simulink model "Figure_2_4_TP_Modulation_phase_quadrature"  (R2020a)
settings: Solver=FixedStepDiscrete  StartTime=0.0  StopTime=inf  RelTol=1e-3
libraries: dspsrcs4 x5, commutil2 x4, simulink x3, commrandsrc3 x2, commfilt2 x2, commsink2 x1
settings Model: Creator=iba  LastModifiedBy=iba

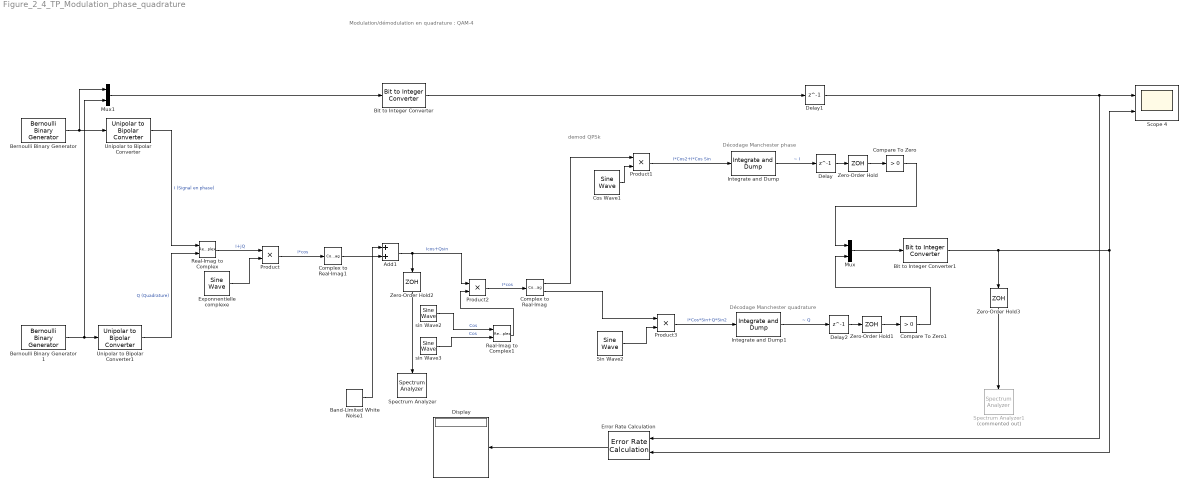
== system Figure_2_4_TP_Modulation_phase_quadrature ==
  note: Décodage Manchester phase
  note: Décodage Manchester quadrature
  note: demod QPSk
  note: Modulation/démodulation en quadrature : QAM-4
  Add1 : Sum
  Band-Limited White Noise1 : simulink/Sources/Band-Limited White Noise  Cov=1e-3  Ts=0.1  seed=1
  "Bernoulli Binary Generator " : commrandsrc3/Bernoulli Binary Generator  ProbabilityOfZero=0.5  SeedSource=Parameter  Seed=61  SampleTime=1  SamplesPerFrame=1  OutputDataType=double  SimulateUsing=Interpreted execution
  Bernoulli Binary Generator 1 : commrandsrc3/Bernoulli Binary Generator  ProbabilityOfZero=0.5  SeedSource=Parameter  Seed=23  SampleTime=1  SamplesPerFrame=1  OutputDataType=double  SimulateUsing=Interpreted execution
  Bit to Integer Converter : commutil2/Bit to Integer Converter  nbits=2  bitOrder=MSB first  signedOutputValues=Unsigned  outDtype=double  outDtypeSigned=Inherit via internal rule
  Bit to Integer Converter1 : commutil2/Bit to Integer Converter  nbits=2  bitOrder=MSB first  signedOutputValues=Unsigned  outDtype=double  outDtypeSigned=Inherit via internal rule
  Compare To Zero : simulink/Logic and Bit Operations/Compare To Zero  relop=>  OutDataTypeStr=boolean
  Compare To Zero1 : simulink/Logic and Bit Operations/Compare To Zero  relop=>  OutDataTypeStr=boolean
  Complex to Real-Imag : ComplexToRealImag
  Complex to Real-Imag1 : ComplexToRealImag  Output=Real
  Cos Wave1 : dspsrcs4/Sine Wave  Amplitude=1  Frequency=5  Phase=pi/2  SampleMode=Discrete  OutComplex=Real  CompMethod=Trigonometric fcn  TableSize=Speed  SampleTime=1/100  SamplesPerFrame=1  ResetState=Restart at time zero  OutputFrames=off  dataType=double  wordLen=16  udDataType=sfix(16)  fracBitsMode=Best precision  numFracBits=15  OutDataTypeStr=double  LastOutDataTypeStr=double
  Delay : Delay  DelayLength=1  InitialCondition=0
  Delay1 : Delay  DelayLength=1  InitialCondition=0
  Delay2 : Delay  DelayLength=1  InitialCondition=0
  Display : Display
  Error Rate Calculation : commsink2/Error Rate Calculation  N=0  st_delay=0  cp_mode=Entire frame  subframe=[]  PMode=Port  WsName=ErrorVec  RsMode2=off  stop=on  numErr=1000  maxBits=1000
  Exponnentielle complexe : dspsrcs4/Sine Wave  Amplitude=exp(1)  Frequency=5  Phase=0  SampleMode=Discrete  OutComplex=Real  CompMethod=Trigonometric fcn  TableSize=Speed  SampleTime=1/100  SamplesPerFrame=1  ResetState=Restart at time zero  OutputFrames=off  dataType=double  wordLen=16  udDataType=sfix(16)  fracBitsMode=Best precision  numFracBits=15  OutDataTypeStr=double  LastOutDataTypeStr=double
  Integrate and Dump : commfilt2/Integrate and Dump  obssamples=100  offsetsamples=0  nodump=on  roundingMode=Floor  overflowMode=off  outputDataTypeStr=Inherit: Same as accumulator  outputLastDataTypeStr=Inherit: Same as accumulator
  Integrate and Dump1 : commfilt2/Integrate and Dump  obssamples=100  offsetsamples=0  nodump=on  roundingMode=Floor  overflowMode=off  outputDataTypeStr=Inherit: Same as accumulator  outputLastDataTypeStr=Inherit: Same as accumulator
  Mux : Mux  Inputs=2
  Mux1 : Mux  Inputs=2
  Product{,1..3} (4 alike) : Product
  Real-Imag to Complex : RealImagToComplex
  Real-Imag to Complex1 : RealImagToComplex
  Scope 4 : Scope  NumInputPorts=2
  Sin Wave2 : dspsrcs4/Sine Wave  Amplitude=1  Frequency=5  Phase=0  SampleMode=Discrete  OutComplex=Real  CompMethod=Trigonometric fcn  TableSize=Speed  SampleTime=1/100  SamplesPerFrame=1  ResetState=Restart at time zero  OutputFrames=off  dataType=double  wordLen=16  udDataType=sfix(16)  fracBitsMode=Best precision  numFracBits=15  OutDataTypeStr=double  LastOutDataTypeStr=double
  Spectrum Analyzer : SpectrumAnalyzer
  Spectrum Analyzer1 : SpectrumAnalyzer  Commented=on
  Unipolar to Bipolar Converter : commutil2/Unipolar to Bipolar Converter  M=2  polarity=Positive  dataType=Inherit via internal rule
  Unipolar to Bipolar Converter1 : commutil2/Unipolar to Bipolar Converter  M=2  polarity=Positive  dataType=Inherit via internal rule
  Zero-Order Hold : ZeroOrderHold
  Zero-Order Hold1 : ZeroOrderHold
  Zero-Order Hold2 : ZeroOrderHold  SampleTime=1/20
  Zero-Order Hold3 : ZeroOrderHold  SampleTime=1/20
  sin Wave2 : dspsrcs4/Sine Wave  Amplitude=1  Frequency=5  Phase=0  SampleMode=Discrete  OutComplex=Real  CompMethod=Trigonometric fcn  TableSize=Speed  SampleTime=1/100  SamplesPerFrame=1  ResetState=Restart at time zero  OutputFrames=off  dataType=double  wordLen=16  udDataType=sfix(16)  fracBitsMode=Best precision  numFracBits=15  OutDataTypeStr=double  LastOutDataTypeStr=double
  sin Wave3 : dspsrcs4/Sine Wave  Amplitude=1  Frequency=5  Phase=0  SampleMode=Discrete  OutComplex=Real  CompMethod=Trigonometric fcn  TableSize=Speed  SampleTime=1/100  SamplesPerFrame=1  ResetState=Restart at time zero  OutputFrames=off  dataType=double  wordLen=16  udDataType=sfix(16)  fracBitsMode=Best precision  numFracBits=15  OutDataTypeStr=double  LastOutDataTypeStr=double
  wires:
  Unipolar to Bipolar Converter/1 -> Real-Imag to Complex/1  "I (Signal en phase)"
  Exponnentielle complexe/1 -> Product/2
  "Bernoulli Binary Generator "/1 -> Mux1/1, Unipolar to Bipolar Converter/1
  Unipolar to Bipolar Converter1/1 -> Real-Imag to Complex/2  "Q (Quadrature)"
  Bernoulli Binary Generator 1/1 -> Mux1/2, Unipolar to Bipolar Converter1/1
  Mux1/1 -> Bit to Integer Converter/1
  Bit to Integer Converter/1 -> Delay1/1
  Bit to Integer Converter1/1 -> Zero-Order Hold3/1, Scope 4/2, Error Rate Calculation/2
  Error Rate Calculation/1 -> Display/1
  Add1/1 -> Product2/1, Zero-Order Hold2/1  "Icos+Qsin"
  Band-Limited White Noise1/1 -> Add1/1
  Compare To Zero1/1 -> Mux/2
  Mux/1 -> Bit to Integer Converter1/1
  Compare To Zero/1 -> Mux/1
  Delay/1 -> Zero-Order Hold/1
  Zero-Order Hold/1 -> Compare To Zero/1
  Integrate and Dump/1 -> Delay/1  "~ I"
  Product3/1 -> Integrate and Dump1/1  "I*Cos*Sin+Q*Sin2"
  Cos Wave1/1 -> Product1/2
  Delay2/1 -> Zero-Order Hold1/1
  Product1/1 -> Integrate and Dump/1  "I*Cos2+I*Cos Sin"
  Sin Wave2/1 -> Product3/2
  Zero-Order Hold1/1 -> Compare To Zero1/1
  Integrate and Dump1/1 -> Delay2/1  "~ Q"
  Zero-Order Hold2/1 -> Spectrum Analyzer/1
  Zero-Order Hold3/1 -> Spectrum Analyzer1/1
  Delay1/1 -> Error Rate Calculation/1, Scope 4/1
  Product/1 -> Complex to Real-Imag1/1  "I*cos"
  Complex to Real-Imag1/1 -> Add1/2
  Real-Imag to Complex/1 -> Product/1  "I+jQ"
  sin Wave3/1 -> Real-Imag to Complex1/2  "Cos"
  sin Wave2/1 -> Real-Imag to Complex1/1  "Cos"
  Real-Imag to Complex1/1 -> Product2/2
  Product2/1 -> Complex to Real-Imag/1  "I*cos"
  Complex to Real-Imag/2 -> Product3/1
  Complex to Real-Imag/1 -> Product1/1
